simulink model "setHoming"  (R2016a)
settings: Solver=FixedStepDiscrete  StartTime=0.0  StopTime=inf  FixedStep=0.008  RelTol=1e-3
PreLoadFcn:
  | if ~exist('Ts', 'var')
  | Ts = 0.001;
  | end
  | if ~exist('Tpwm', 'var')
  | Tpwm = 0.005;
  | end
  | if ~exist('FPGA_Frequency', 'var')
  | FPGA_Frequency = 75000000;
  | end
undefined symbols (not defined in the file or in its folder): IO3xx
libraries: speedgoatlib_fpga x6, slrtlib x4
settings Model: Creator=cedric  LastModifiedBy=kqp5516
settings SolverCC: EnableConcurrentExecution=on
settings DataIOCC: SaveFormat=StructureWithTime
settings OptimizationCC: BlockReduction=off  OptimizeBlockIOStorage=off  BufferReuse=off  GlobalBufferReuse=off  ExpressionFolding=off  LocalBlockOutputs=off
settings DebuggingCC: UnderspecifiedInitializationDetection=Classic  MergeDetectMultiDrivingBlocksExec=none  UnconnectedInputMsg=none  UnconnectedOutputMsg=none  UnconnectedLineMsg=none  SFUnexpectedBacktrackingDiag=error  SFNoUnconditionalDefaultTransitionDiag=error
settings HardwareCC: ProdBitPerPointer=32  ProdLargestAtomicFloat=None  ProdWordSize=32  ProdHWDeviceType=Generic->32-bit x86 compatible
settings ModelReferenceCC: PropagateSignalLabelsOutOfModel=off
settings RTWCC: SystemTargetFile=slrt.tlc  TemplateMakefile=slrt_default_tmf  Description=Simulink Real-Time  RTWCompilerOptimization=on
settings SimulinkRealTimeCC: RL32LogTETModifier=off  xPCisModelTimeout=off  xPCModelTimeoutSecs=20
settings ConfigComp: CovMetricSettings=dwe  CovHtmlReporting=off  CovSaveCumulativeToWorkspaceVar=off  CovSaveSingleToWorkspaceVar=off  CovExternalEMLEnable=on

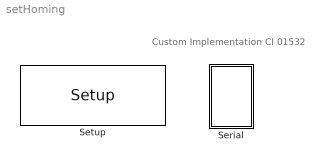
== system setHoming ==
  note: Custom Implementation CI 01532
  Serial : Subsystem
  Setup : speedgoatlib_fpga/Setup/Setup  board=IO323  id=1  frontIO=None  rearIO=IO3xx-22  bitstreamFile=speedgoat_IO323_22_CI_01532  ProgSpiFlash=off  ProgBPIFlash=off  pciSlot=-1  PullRPort0=pull-up 3.3V  VioPort0=3.3V  PullRPort1=pull-up 3.3V  VioPort1=3.3V  PullRPort2=pull-up 3.3V  VioPort2=3.3V  PullRPort3=pull-up 3.3V  VioPort3=3.3V  PullRPort4=pull-up 3.3V  VioPort4=3.3V  PullRPort5=pull-up 3.3V  VioPort5=3.3V  PullRPort6=pull-up 3.3V  VioPort6=3.3V  PullRPort15=pull-up 3.3V  PullRPort31=pull-up 3.3V  PullRPort47=pull-up 3.3V  PullRPort63=pull-up 3.3V

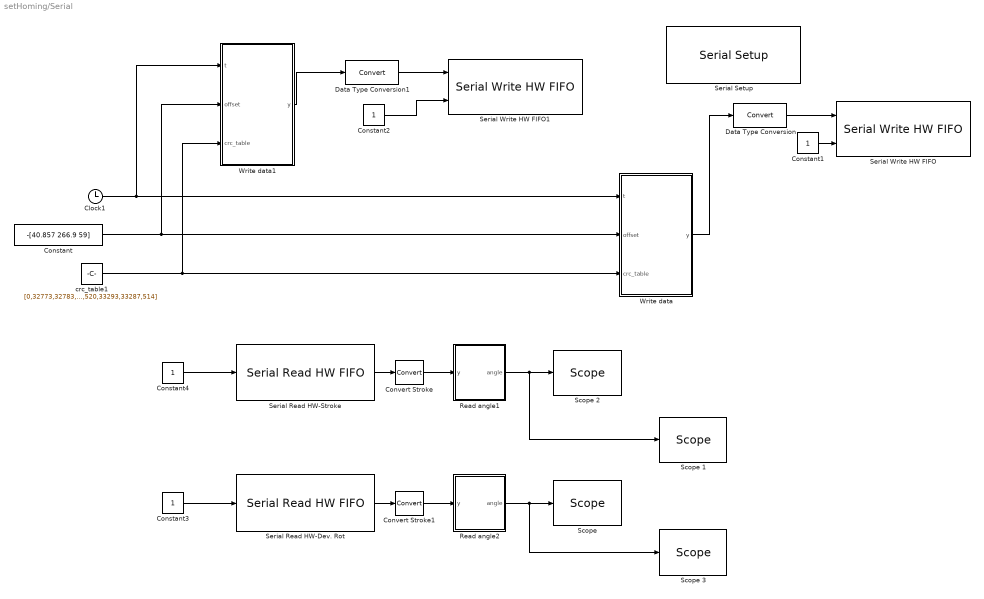
== system setHoming/Serial ==
  Clock1 : Clock
  Constant : Constant  Value=-[40.857 266.9 59]
  Constant{1..4} (4 alike) : Constant  OutDataTypeStr=Inherit: Inherit via back propagation
  Convert Stroke : DataTypeConversion
  Convert Stroke1 : DataTypeConversion
  Data Type Conversion : DataTypeConversion
  Data Type Conversion1 : DataTypeConversion
  Read angle1 : MATLAB Function  TreatAsAtomicUnit=on
  Read angle2 : MATLAB Function  TreatAsAtomicUnit=on
  "Scope " : slrtlib/Displays and Logging/Scope   scopeno=2  scopetype=Target  autostart=on  viewmode=Numerical  formatstr='%15.6f'  grid=on  ylimits=[0,0]  nosamples=100  noprepostsamples=0  interleave=1  triggermode=FreeRun  triggersignal=1  trigsignalfromport=off  triggerlevel=0.0  triggerslope=Either  triggerscope=1  triggersample=0  filename=data.dat  mode=Lazy  writesize=512  autorestart=off  dynamicfilemode=off  maxwritefilesize=512*1024^2
  Scope 1 : slrtlib/Displays and Logging/Scope   scopeno=3  scopetype=Target  autostart=on  viewmode=Graphical rolling  formatstr='%15.6f'  grid=on  ylimits=[-90,90]  nosamples=500  noprepostsamples=0  interleave=1  triggermode=FreeRun  triggersignal=1  trigsignalfromport=off  triggerlevel=0.0  triggerslope=Either  triggerscope=1  triggersample=0  filename=data.dat  mode=Lazy  writesize=512  autorestart=off  dynamicfilemode=off  maxwritefilesize=512*1024^2
  Scope 2 : slrtlib/Displays and Logging/Scope   scopeno=1  scopetype=Target  autostart=on  viewmode=Numerical  formatstr='%15.6f'  grid=on  ylimits=[0,0]  nosamples=100  noprepostsamples=0  interleave=1  triggermode=FreeRun  triggersignal=1  trigsignalfromport=off  triggerlevel=0.0  triggerslope=Either  triggerscope=1  triggersample=0  filename=data.dat  mode=Lazy  writesize=512  autorestart=off  dynamicfilemode=off  maxwritefilesize=512*1024^2
  Scope 3 : slrtlib/Displays and Logging/Scope   scopeno=4  scopetype=Target  autostart=on  viewmode=Graphical rolling  formatstr='%15.6f'  grid=on  ylimits=[-30,100]  nosamples=500  noprepostsamples=0  interleave=1  triggermode=FreeRun  triggersignal=1  trigsignalfromport=off  triggerlevel=0.0  triggerslope=Either  triggerscope=1  triggersample=0  filename=data.dat  mode=Lazy  writesize=512  autorestart=off  dynamicfilemode=off  maxwritefilesize=512*1024^2
  Serial Read HW-Dev. Rot : speedgoatlib_fpga/Serial/Serial Read HW FIFO  id=1  channel=6  board=IO323  nb_data_bits=8  pciSlot=-1  ts=0.008
  Serial Read HW-Stroke : speedgoatlib_fpga/Serial/Serial Read HW FIFO  id=1  channel=1  board=IO323  nb_data_bits=8  pciSlot=-1  ts=0.008
  Serial Setup : speedgoatlib_fpga/Serial/Serial Setup  id=1  channel=[1 6]  bitrate_configuration=Simple  bitrate=[1000000]  bitrate_effective=[1e6, 1e6]  bitrate_error=[0, 0]  base_clock=[75000000, 75000000]  divider=[5, 5]  cpr=[1, 1]  tcr=[15, 15]  parity=No parity  nb_data_bits=[8]  nb_stop_bits=[1]  rs485_half_duplex=on  board=IO323  pciSlot=-1
  Serial Write HW FIFO : speedgoatlib_fpga/Serial/Serial Write HW FIFO  id=1  channel=1  board=IO323  tx_fifo_mode=Halt model on buffer overflow  nb_data_bits=8  pciSlot=-1  ts=0.008
  Serial Write HW FIFO1 : speedgoatlib_fpga/Serial/Serial Write HW FIFO  id=1  channel=6  board=IO323  tx_fifo_mode=Halt model on buffer overflow  nb_data_bits=8  pciSlot=-1  ts=0.008
  Write data : MATLAB Function  TreatAsAtomicUnit=on
  Write data1 : MATLAB Function  TreatAsAtomicUnit=on
  crc_table1 : Constant  Value=[0,32773,32783,10,32795,30,20,32785,32819,54,60,32825,40,32813,32807,34,32867,102,108,32873,120,32893,32887,114,80,32853,32863,90,32843,78,68,32833,32963,198,204,32969,216,32989,32983,210,240,33013,33023,250,33003,238,228,32993,160,32933,32943,170,32955,190,180,32945,32915,150,156,32921,136,32909,32903,130,33155,390,396,33161,408,33181,33175,402,432,33205,33215,442,33195,430,420,33185,480,33253,33263,490,33275,510,500,33265,33235,470,476,33241,456,33229,33223,450,320,33093,33103,330,33115,350,340,33105,33139,374,380,33145,360,33133,33127,354,33059,294,300,33065,312,33085,33079,306,272,33045,33055,282,33035,270,260,33025,33539,774,780,33545,792,33565,33559,786,816,33589,33599,826,33579,814,804,33569,864,33637,33647,874,33659,894,884,33649,33619,854,860,33625,840,33613,33607,834,960,33733,33743,970,33755,990,980,33745,33779,1014,1020,33785,1000,33773,33767,994,33699,934,940,33705,952,33725,33719,946,912,33685,33695,922,33675,910,900,33665,640,33413,33423,650,33435,670,660,33425,33459,694,700,33465,680,33453,33447,674,33507,742,748,33513,760,33533,33527,754,720,33493,33503,730,33483,718,708,33473,33347,582,588,33353,600,33373,33367,594,624,33397,33407,634,33387,622,612,33377,544,33317,33327,554,33339,574,564,33329,33299,534,540,33305,520,33293,33287,514]  OutDataTypeStr=Inherit: Inherit via back propagation
  wires:
  Constant1/1 -> Serial Write HW FIFO/2
  Data Type Conversion/1 -> Serial Write HW FIFO/1
  Write data/1(y) -> Data Type Conversion/1
  Constant2/1 -> Serial Write HW FIFO1/2
  Clock1/1 -> Write data/1(t), Write data1/1(t)
  Data Type Conversion1/1 -> Serial Write HW FIFO1/1
  crc_table1/1 -> Write data1/3(crc_table), Write data/3(crc_table)
  Constant3/1 -> Serial Read HW-Dev. Rot/1
  Constant4/1 -> Serial Read HW-Stroke/1
  Serial Read HW-Stroke/1 -> Convert Stroke/1
  Serial Read HW-Dev. Rot/1 -> Convert Stroke1/1
  Read angle1/1(angle) -> Scope 1/1, Scope 2/1
  Convert Stroke/1 -> Read angle1/1(y)
  Convert Stroke1/1 -> Read angle2/1(y)
  Read angle2/1(angle) -> Scope 3/1, "Scope "/1
  Write data1/1(y) -> Data Type Conversion1/1
  Constant/1 -> Write data1/2(offset), Write data/2(offset)

== matlab function setHoming/Serial/Write data ==
  data: y output; t input; offset input; crc_table input
function y = fcn(t,offset,crc_table)
%#codegen

% do the following on BOTH scripts
% step 1: make offset = -[0 0 0] and upload to Speedgoat
% step 2: put robot at home position
% step 3: read angles from Speedgoat monitor
% step 4: make offset = -[angles from speedgoat]
% step 5: reupload

if t == 0.0     % initialization
    y = packetMultiWrite(3,[1 2 3],[0 0 0],crc_table);
elseif t<0.1
    %% WRITE
    % offset = -[63.91 59.96 -30.4];
    y = packetMultiWrite(20,[1 2 3], offset, crc_table);
    
else
    %% READ
    y = packetMultiWrite(13,1,[1 1 1],crc_table);
end

end

== matlab function setHoming/Serial/Write data1 ==
  data: y output; t input; offset input; crc_table input
function y = fcn(t,offset,crc_table)
%#codegen

% do the following on BOTH scripts
% step 1: make offset = -[0 0 0] and upload to Speedgoat
% step 2: put robot at home position
% step 3: read angles from Speedgoat monitor
% step 4: make offset = -[angles from speedgoat]
% step 5: reupload

if t == 0.0     % initialization
    y = packetMultiWrite(3,[1 2 3],[0 0 0],crc_table);
elseif t<0.1
    %% WRITE
    % offset = -[63.91 59.96 -30.4];
    y = packetMultiWrite(20,[1 2 3], offset, crc_table);
    
else
    %% READ
    y = packetMultiWrite(14,[1 2 3],[1 1 1],crc_table);
end

end

== matlab function setHoming/Serial/Read angle1 ==
  data: y input; angle output
function angle  = fcn(y)
%#codegen
angle = 0;
ID = 1;
Negative_allowed = 1;
for i = 1:1:length(y)-5
    if y(i) == 255 && y(i+1) == 255 && y(i+2) == 253 && y(i+4) == ID && y(i+5) == 8
        temp = i;
        Para = y(temp+9:temp+12);
        angle = Position(Para,Negative_allowed);
    end
end

end

function angle = Position(para,Neg_allowed)

switch(Neg_allowed)
    case 0
        value_byte = double(typecast(uint8(para),'uint32'));
    case 1
        value_byte = double(typecast(uint8(para),'int32'));
end

angle = value_byte*360/4095;
end

== matlab function setHoming/Serial/Read angle2 ==
  data: y input; angle output size=[1 2]
function angle  = fcn(y)
%#codegen

angle_2 = 0;
angle_3 = 0;
ID = [2 3];
for i = 1:1:length(y)-5
    if y(i) == 255 && y(i+1) == 255 && y(i+2) == 253 && y(i+4) == ID(1) && y(i+5) == 8
        temp_2 = i;
        Para_2 = y(temp_2+9:temp_2+12);
        angle_2 = Position(Para_2);
    elseif y(i) == 255 && y(i+1) == 255 && y(i+2) == 253 && y(i+4) == ID(2) && y(i+5) == 8
        temp_3 = i;
        Para_3 = y(temp_3+9:temp_3+12);
        angle_3 = Position(Para_3);
    end
end
angle = [angle_2 angle_3];
end

function angle = Position(para)
value_byte = double(typecast(uint8(para),'int32'));
angle = value_byte*360/4095;
end
